simulink model "MBD_ques2"  (R2020a)
settings: Solver=VariableStepAuto  StartTime=0.0  StopTime=100  RelTol=1e-3
settings Model: Creator=DELL  LastModifiedBy=DELL

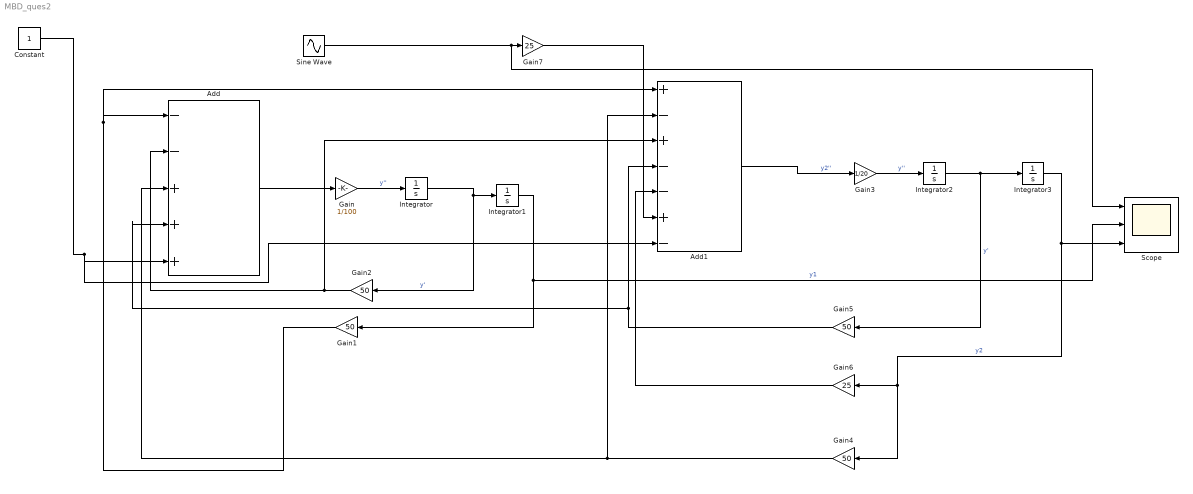
== system MBD_ques2 ==
  Add : Sum  Inputs=--+++
  Add1 : Sum  Inputs=+-+--+-
  Constant : Constant
  Gain : Gain  Gain=1/100
  Gain{1..2,4..5} (4 alike) : Gain  Gain=50
  Gain3 : Gain  Gain=1/20
  Gain6 : Gain  Gain=25
  Gain7 : Gain  Gain=25
  Integrator{,1..3} (4 alike) : Integrator
  Scope : Scope  NumInputPorts=3
  Sine Wave : Sin  Amplitude=2  Frequency=10  SampleTime=0
  wires:
  Add/1 -> Gain/1
  Gain/1 -> Integrator/1  "y''"
  Integrator/1 -> Integrator1/1, Gain2/1  "y'"
  Integrator1/1 -> Gain1/1, Scope/2  "y1"
  Gain1/1 -> Add1/1, Add/1
  Gain2/1 -> Add1/3, Add/2
  Add1/1 -> Gain3/1  "y2''"
  Gain3/1 -> Integrator2/1  "y''"
  Integrator2/1 -> Gain5/1, Integrator3/1  "y'"
  Integrator3/1 -> Gain6/1, Gain4/1, Scope/3  "y2"
  Gain4/1 -> Add/3, Add1/2
  Gain5/1 -> Add/4, Add1/4
  Gain6/1 -> Add1/5
  Sine Wave/1 -> Scope/1, Gain7/1
  Gain7/1 -> Add1/6
  Constant/1 -> Add1/7, Add/5
